simulink model "bislip_sim"  (R2015b)
settings: Solver=FixedStepAuto  StartTime=0.0  StopTime=100  FixedStep=Ts/16  MaxStep=Ts  MinStep=Ts/4  RelTol=1e-3
values from neighbouring files (symbols this model uses):
  a = 2*pi*freq*obj.Ts/(2*pi*freq*obj.Ts + 1)    [StateEstimator.m]
  ground_data = zeros(2, 5)    [BipedVisualization.m]    (also in Planner.m; biped_setup.m = [ground_x, ground_y, ground_stiffness, ground_damping, groun)
  params = zeros(11, 1)    [DoubleSupportController.m]    (also in FlightController.m; LegController.m; PlanarBipedController.m = zeros(12, 1); Sequencing.m)
  Ts = 1e-3    (= 0.001)    [BipedController.m]    (also in Planner.m = 0.1; Sequencing.m; StateEstimator.m)
  X0 = struct()    [RobotState.m]    (also in biped_setup.m = RobotState())
undefined symbols (not defined in the file or in its folder): body_mass, foot_mass, gravity, leg_stiffness
settings Model: Creator=patrick  LastModifiedBy=robots
settings SolverCC: InitialStep=Ts

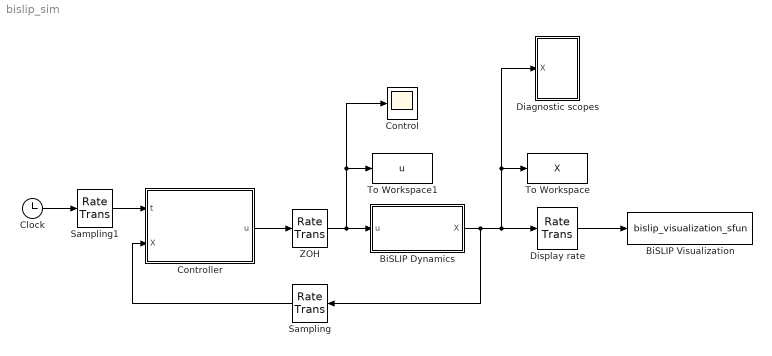
== system bislip_sim ==
  BiSLIP Dynamics : Subsystem  mask{Y0=X0, params=params, ground_data=ground_data}
      mask prompts: Y0 "Initial states:"; params "Model parameters:"; ground_data "Ground data:"
      mask DialogControl DescTextVar Prompt: BiSLIP system dynamics
      mask Display:
      | port_label('input', 1, 'u')
      | port_label('output', 1, 'X')
  BiSLIP Visualization : M-S-Function  FunctionName=bislip_visualization_sfun  Parameters=ground_data
  Clock : Clock
  Control : Scope
  Controller : Subsystem
  Diagnostic scopes : Subsystem
  Display rate : RateTransition  OutPortSampleTime=Ts*6
  Sampling : RateTransition  OutPortSampleTime=Ts
  Sampling1 : RateTransition  OutPortSampleTime=Ts
  To Workspace : ToWorkspace  VariableName=X  SaveFormat=Timeseries  SampleTime=-1
  To Workspace1 : ToWorkspace  VariableName=u  SaveFormat=Timeseries  SampleTime=-1
  ZOH : RateTransition  OutPortSampleTimeOpt=Inherit  OutPortSampleTime=-a
  wires:
  ZOH/1 -> BiSLIP Dynamics/1(u), Control/1, To Workspace1/1
  Controller/1(u) -> ZOH/1
  BiSLIP Dynamics/1(X) -> Diagnostic scopes/1(X), To Workspace/1, Display rate/1, Sampling/1
  Display rate/1 -> BiSLIP Visualization/1
  Sampling/1 -> Controller/2(X)
  Clock/1 -> Sampling1/1
  Sampling1/1 -> Controller/1(t)

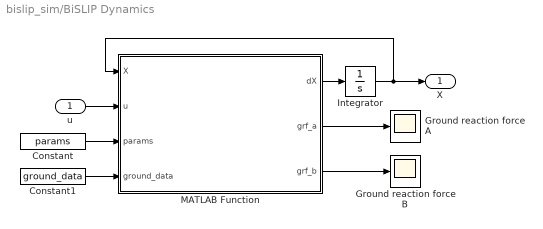
== system bislip_sim/BiSLIP Dynamics ==
  u : Inport
  Constant : Constant  Value=params
  Constant1 : Constant  Value=ground_data
  Ground reaction force A : Scope
  Ground reaction force B : Scope
  Integrator : Integrator  InitialCondition=X0
  MATLAB Function : MATLAB Function  TreatAsAtomicUnit=on
  X : Outport
  wires:
  Integrator/1 -> X/1, MATLAB Function/1(X)
  u/1 -> MATLAB Function/2(u)
  Constant/1 -> MATLAB Function/3(params)
  Constant1/1 -> MATLAB Function/4(ground_data)
  MATLAB Function/1(dX) -> Integrator/1
  MATLAB Function/2(grf_a) -> Ground reaction force A/1
  MATLAB Function/3(grf_b) -> Ground reaction force B/1

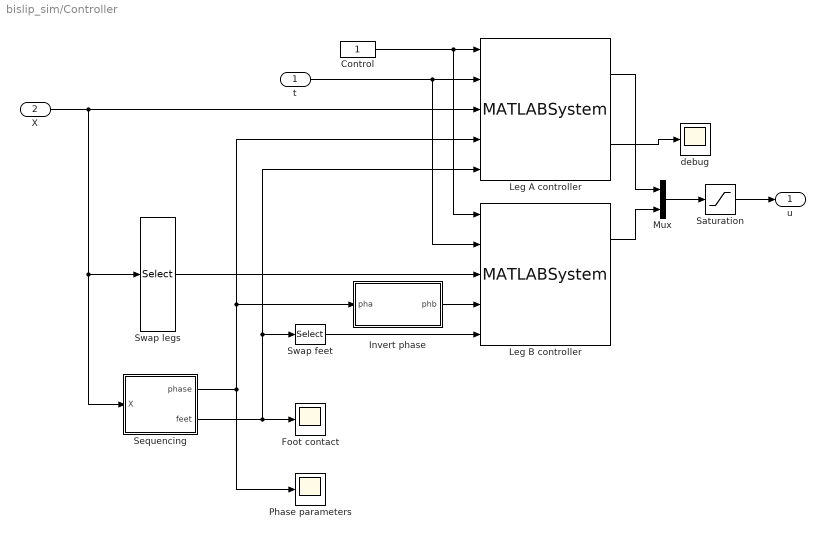
== system bislip_sim/Controller ==
  t : Inport
  X : Inport  Port=2
  Control : Constant
  Foot contact : Scope
  Invert phase : MATLAB Function  TreatAsAtomicUnit=on
  Leg A controller : MATLABSystem  System=LegController  params=params  SimulateUsing=Interpreted execution
      mask Type: LegController
      mask Display:
      | disp('LegController');
      | port_label('input',1,'control');
      | port_label('input',2,'t');
      | port_label('input',3,'X');
      | port_label('input',4,'phase');
      | port_label('input',5,'feet');
      | port_label('output',1,'u');
      | port_label('output',2,'debug');
  Leg B controller : MATLABSystem  System=LegController  params=params  SimulateUsing=Interpreted execution
      mask Type: LegController
      mask Display:
      | disp('LegController');
      | port_label('input',1,'control');
      | port_label('input',2,'t');
      | port_label('input',3,'X');
      | port_label('input',4,'phase');
      | port_label('input',5,'feet');
      | port_label('output',1,'u');
      | port_label('output',2,'debug');
  Mux : Mux  Inputs=2
  Phase parameters : Scope
  Saturation : Saturate  UpperLimit=[1e4 1e3 1e4 1e3]  LowerLimit=-[1e4 1e3 1e4 1e3]
  Sequencing : Subsystem
  Swap feet : Selector  InputPortWidth=2  IndexOptions=Index vector (dialog)  Indices=[2 1]  OutputSizes=1
  Swap legs : Selector  InputPortWidth=18  IndexOptions=Index vector (dialog)  Indices=[1:6 13:18 7:12]  OutputSizes=1
  debug : Scope
  u : Outport
  wires:
  X/1 -> Leg A controller/3, Sequencing/1(X), Swap legs/1
  Control/1 -> Leg B controller/1, Leg A controller/1
  Swap legs/1 -> Leg B controller/3
  t/1 -> Leg B controller/2, Leg A controller/2
  Sequencing/1(phase) -> Leg A controller/4, Invert phase/1(pha), Phase parameters/1
  Swap feet/1 -> Leg B controller/5
  Invert phase/1(phb) -> Leg B controller/4
  Leg A controller/1 -> Mux/1
  Leg B controller/1 -> Mux/2
  Mux/1 -> Saturation/1
  Sequencing/2(feet) -> Leg A controller/5, Swap feet/1, Foot contact/1
  Saturation/1 -> u/1
  Leg A controller/2 -> debug/1

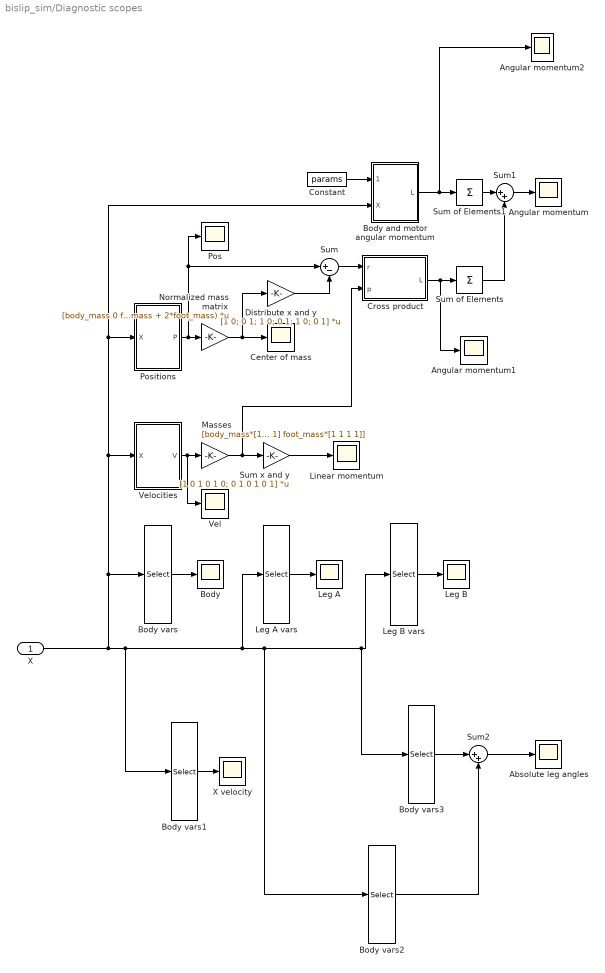
== system bislip_sim/Diagnostic scopes ==
  X : Inport
  Absolute leg angles : Scope
  Angular momentum : Scope
  Angular momentum1 : Scope
  Angular momentum2 : Scope
  Body : Scope
  Body and motor angular momentum : MATLAB Function  TreatAsAtomicUnit=on
  Body vars : Selector  InputPortWidth=18  IndexOptions=Index vector (dialog)  Indices=[1:6]  OutputSizes=1
  Body vars1 : Selector  InputPortWidth=18  IndexOptions=Index vector (dialog)  Indices=[2]  OutputSizes=1
  Body vars2 : Selector  InputPortWidth=18  IndexOptions=Index vector (dialog)  Indices=[5]  OutputSizes=1
  Body vars3 : Selector  InputPortWidth=18  IndexOptions=Index vector (dialog)  Indices=[11 17]  OutputSizes=1
  Center of mass : Scope
  Constant : Constant  Value=params
  Cross product : MATLAB Function  TreatAsAtomicUnit=on
  Distribute x and y : Gain  Gain=[1 0; 0 1; 1 0; 0 1; 1 0; 0 1]  Multiplication=Matrix(K*u)
  Leg A : Scope
  Leg A vars : Selector  InputPortWidth=18  IndexOptions=Index vector (dialog)  Indices=[7:12]  OutputSizes=1
  Leg B : Scope
  Leg B vars : Selector  InputPortWidth=18  IndexOptions=Index vector (dialog)  Indices=[13:18]  OutputSizes=1
  Linear momentum : Scope
  Masses : Gain  Gain=[body_mass*[1 1] foot_mass*[1 1 1 1]]
  Normalized mass matrix : Gain  Gain=[body_mass 0 foot_mass 0 foot_mass 0; 0 body_mass 0 foot_mass 0 foot_mass]/(body_mass + 2*foot_mass)  Multiplication=Matrix(K*u)
  Pos : Scope
  Positions : MATLAB Function  TreatAsAtomicUnit=on
  Sum : Sum  Inputs=|+-
  Sum of Elements : Sum  Inputs=+
  Sum of Elements1 : Sum  Inputs=+
  Sum x and y : Gain  Gain=[1 0 1 0 1 0; 0 1 0 1 0 1]  Multiplication=Matrix(K*u)
  Sum1 : Sum  Inputs=|++
  Sum2 : Sum  Inputs=|++
  Vel : Scope
  Velocities : MATLAB Function  TreatAsAtomicUnit=on
  X velocity : Scope
  wires:
  Positions/1(P) -> Sum/1, Pos/1, Normalized mass matrix/1
  Normalized mass matrix/1 -> Center of mass/1, Distribute x and y/1
  Sum of Elements/1 -> Sum1/2
  Sum/1 -> Cross product/1(r)
  Sum1/1 -> Angular momentum/1
  Body vars/1 -> Body/1
  Masses/1 -> Cross product/2(p), Sum x and y/1
  Leg B vars/1 -> Leg B/1
  Leg A vars/1 -> Leg A/1
  Velocities/1(V) -> Vel/1, Masses/1
  Distribute x and y/1 -> Sum/2
  Cross product/1(L) -> Angular momentum1/1, Sum of Elements/1
  Sum x and y/1 -> Linear momentum/1
  Body and motor angular momentum/1(L) -> Angular momentum2/1, Sum of Elements1/1
  X/1 -> Body vars1/1, Body vars2/1, Body vars3/1, Leg B vars/1, Leg A vars/1, Velocities/1(X), Body and motor angular momentum/2(X), Positions/1(X), Body vars/1
  Sum of Elements1/1 -> Sum1/1
  Constant/1 -> Body and motor angular momentum/1(params)
  Body vars1/1 -> X velocity/1
  Body vars3/1 -> Sum2/1
  Body vars2/1 -> Sum2/2
  Sum2/1 -> Absolute leg angles/1

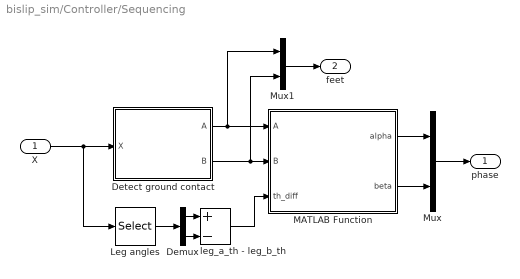
== system bislip_sim/Controller/Sequencing ==
  X : Inport
  Demux : Demux  Outputs=2
  Detect ground contact : Subsystem
  Leg angles : Selector  InputPortWidth=18  IndexOptions=Index vector (dialog)  Indices=[11 17]  OutputSizes=1
  MATLAB Function : MATLAB Function  TreatAsAtomicUnit=on
  Mux : Mux  Inputs=2
  Mux1 : Mux  Inputs=2
  leg_a_th - leg_b_th : Sum  Inputs=+-
  phase : Outport
  feet : Outport  Port=2
  wires:
  leg_a_th - leg_b_th/1 -> MATLAB Function/3(th_diff)
  MATLAB Function/2(beta) -> Mux/2
  X/1 -> Leg angles/1, Detect ground contact/1(X)
  MATLAB Function/1(alpha) -> Mux/1
  Detect ground contact/1(A) -> Mux1/1, MATLAB Function/1(A)
  Detect ground contact/2(B) -> Mux1/2, MATLAB Function/2(B)
  Leg angles/1 -> Demux/1
  Demux/1 -> leg_a_th - leg_b_th/1
  Demux/2 -> leg_a_th - leg_b_th/2
  Mux/1 -> phase/1
  Mux1/1 -> feet/1

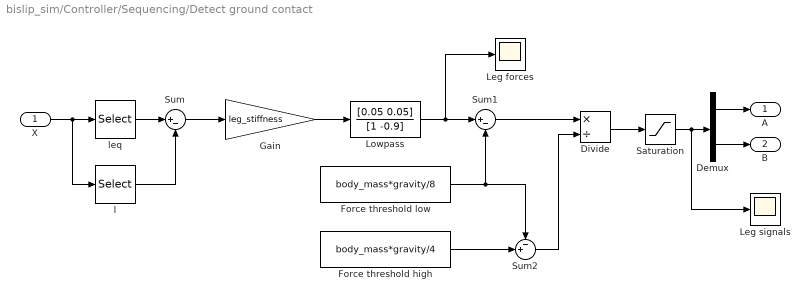
== system bislip_sim/Controller/Sequencing/Detect ground contact ==
  X : Inport
  Demux : Demux  Outputs=2
  Divide : Product  Inputs=*/
  Force threshold high : Constant  Value=body_mass*gravity/4
  Force threshold low : Constant  Value=body_mass*gravity/8
  Gain : Gain  Gain=leg_stiffness
  Leg forces : Scope
  Leg signals : Scope
  Lowpass : DiscreteFilter  Numerator=[0.05 0.05]  Denominator=[1 -0.9]
  Saturation : Saturate  UpperLimit=1  LowerLimit=0
  Sum : Sum  Inputs=|+-
  Sum1 : Sum  Inputs=|+-
  Sum2 : Sum  Inputs=-+|
  l : Selector  InputPortWidth=18  IndexOptions=Index vector (dialog)  Indices=[9 15]  OutputSizes=1
  leq : Selector  InputPortWidth=18  IndexOptions=Index vector (dialog)  Indices=[7 13]  OutputSizes=1
  A : Outport
  B : Outport  Port=2
  wires:
  leq/1 -> Sum/1
  l/1 -> Sum/2
  X/1 -> l/1, leq/1
  Sum/1 -> Gain/1
  Gain/1 -> Lowpass/1
  Divide/1 -> Saturation/1
  Demux/1 -> A/1
  Demux/2 -> B/1
  Saturation/1 -> Leg signals/1, Demux/1
  Sum1/1 -> Divide/1
  Force threshold low/1 -> Sum2/1, Sum1/2
  Force threshold high/1 -> Sum2/2
  Sum2/1 -> Divide/2
  Lowpass/1 -> Leg forces/1, Sum1/1

== matlab function bislip_sim/BiSLIP Dynamics/MATLAB Function ==
  data: X input; u input; dX output; params input; ground_data input; grf_a output; grf_b output
function [dX, grf_a, grf_b] = bislip_dynamics_wrapper(X, u, params, ground_data)
%#codegen

[dX, grf_a, grf_b] = bislip_dynamics(X, u, params, ground_data);

== matlab function bislip_sim/Controller/Sequencing/MATLAB Function ==
  data: A input; B input; th_diff input; alpha output; beta output
function [alpha, beta] = phase_params(A, B, th_diff) %#codegen
% Calculate phase parameters
% alpha: bias towards leg A or leg B, [-1, 1]
% betap: proportion total leg forces, depends on alpha, [0, 1]
% beta: unwrapped betap, [0, 3)
%   0 is flight, A to front
%   1 is double support, A in front
%   2 is flight, B to front
%   3 is double support, B in front

persistent beta_int_last

if isempty(beta_int_last)
    beta_int_last = 0;
end

alpha = (A - B);
if abs(alpha) ~= 1
    betap = (A + B - abs(alpha))/(2*(1 - abs(alpha)));
else
    betap = NaN;
end

if ~isnan(betap)
    switch beta_int_last
        case 0
            if th_diff >= 0
                beta = betap;
            else
                beta = 4 - betap;
            end
        case 1
            beta = 2 - betap;
        case 2
            if th_diff >= 0
                beta = 2 - betap;
            else
                beta = 2 + betap;
            end
        case 3
            beta = 4 - betap;
        otherwise
            error('Invalid value for beta_int_last: %d', beta_int_last);
    end
    beta = mod(beta, 4);
else
    if alpha >= 0
        beta = 2;
    else
        beta = 0;
    end
end
if beta - round(beta) < 1e2*eps(1)
    beta_int_last = mod(round(beta), 4);
end

== matlab function bislip_sim/Diagnostic scopes/Cross product ==
  data: r input; p input; L output
function L = cross(r, p)
%#codegen

L = r(1:2:end).*p(2:2:end) - r(2:2:end).*p(1:2:end);

== matlab function bislip_sim/Diagnostic scopes/Velocities ==
  data: X input; V output
function V = velocities(X) %#codegen
% X: [body_x;    body_xdot;    body_y;  body_ydot;  body_th;  body_thdot;
%     leg_a_leq; leg_a_leqdot; leg_a_l; leg_a_ldot; leg_a_th; leg_a_thdot;
%     leg_b_leq; leg_b_leqdot; leg_b_l; leg_b_ldot; leg_b_th; leg_b_thdot]
% V: [body_xdot; body_ydot; foot_a_xdot; foot_a_ydot; foot_b_xdot; foot_b_ydot]

tha = X(11) + X(5);
thb = X(17) + X(5);
body_vel = X([2 4]);
foot_a_vel = body_vel + X(10)*[sin(tha); -cos(tha)] + (X(12) + X(6))*X(9)*[cos(tha); sin(tha)];
foot_b_vel = body_vel + X(16)*[sin(thb); -cos(thb)] + (X(18) + X(6))*X(15)*[cos(thb); sin(thb)];

V = [body_vel; foot_a_vel; foot_b_vel];

== matlab function bislip_sim/Diagnostic scopes/Positions ==
  data: X input; P output
function P = positions(X) %#codegen
% X: [body_x;    body_xdot;    body_y;  body_ydot;  body_th;  body_thdot;
%     leg_a_leq; leg_a_leqdot; leg_a_l; leg_a_ldot; leg_a_th; leg_a_thdot;
%     leg_b_leq; leg_b_leqdot; leg_b_l; leg_b_ldot; leg_b_th; leg_b_thdot]
% P: [body_x; body_y; foot_a_x; foot_a_y; foot_b_x; foot_b_y]

tha = X(11) + X(5);
thb = X(17) + X(5);
body_pos = X([1 3]);
foot_a_pos = body_pos + X(9)*[sin(tha); -cos(tha)];
foot_b_pos = body_pos + X(15)*[sin(thb); -cos(thb)];

P = [body_pos; foot_a_pos; foot_b_pos];

== matlab function bislip_sim/Diagnostic scopes/Body and motor angular momentum ==
  data: params input; X input; L output
function L = Iw(params, X) %#codegen
% X: [body_x;    body_xdot;    body_y;  body_ydot;  body_th;  body_thdot;
%     leg_a_leq; leg_a_leqdot; leg_a_l; leg_a_ldot; leg_a_th; leg_a_thdot;
%     leg_b_leq; leg_b_leqdot; leg_b_l; leg_b_ldot; leg_b_th; leg_b_thdot]
% P: [body_x; body_y; foot_a_x; foot_a_y; foot_b_x; foot_b_y]

Ib = params(2);
Im = params(8);
n = params(10);

body_w = X(6);
motor_a_w = body_w + n*X(12);
motor_b_w = body_w + n*X(18);

L = [Ib*body_w; Im*motor_a_w; Im*motor_b_w];

== matlab function bislip_sim/Controller/Invert phase ==
  data: pha input; phb output
function phb = invert_phase(pha) %#codegen

phb = [-pha(1); mod(pha(2) + 2, 4)];
